simulink library "DigitalControlLib"  (R2017b)
settings: Solver=VariableStepAuto  StartTime=0.0  StopTime=10.0  RelTol=1e-3
settings Model: Creator=alexandersoussan  LastModifiedBy=alexandersoussan

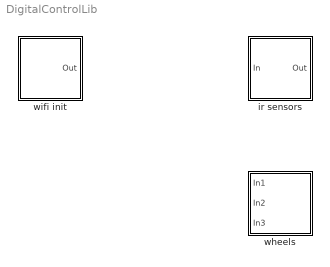
== system DigitalControlLib ==
  ir sensors : Subsystem
  wheels : Subsystem
  wifi init : Subsystem

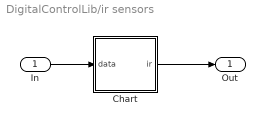
== system DigitalControlLib/ir sensors ==
  In : Inport
  Chart : Stateflow chart  TreatAsAtomicUnit=on
  Out : Outport
  wires:
  Chart/1(ir) -> Out/1
  In/1 -> Chart/1(data)

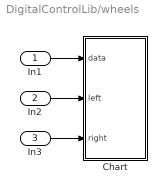
== system DigitalControlLib/wheels ==
  In1 : Inport
  In2 : Inport  Port=2
  In3 : Inport  Port=3
  Chart : Stateflow chart  TreatAsAtomicUnit=on
  wires:
  In1/1 -> Chart/1(data)
  In2/1 -> Chart/2(left)
  In3/1 -> Chart/3(right)

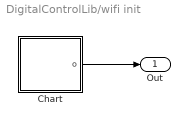
== system DigitalControlLib/wifi init ==
  Chart : Stateflow chart  TreatAsAtomicUnit=on
  Out : Outport
  wires:
  Chart/1(o) -> Out/1

== stateflow chart DigitalControlLib/ir sensors/Chart ==
  state RANGE
    en,du:
    ir=irv;
  (default) -> RANGE
  data: y function_output; ir output; data input
  function y = irv:
    | function y = irv
    | y = [0,0,0,0,0,0];
    | persistent obj
    | coder.extrinsic('evalin')
    | coder.extrinsic('get')
    | coder.extrinsic('RangeStateRoomba')
    | if isempty(obj)
    |     obj = evalin('base','objWs')
    | end
    | coder.extrinsic('RangeStateRoomba')
    | y = RangeStateRoomba(obj);

== stateflow chart DigitalControlLib/wheels/Chart ==
  state Wheels
    en,du:
    wheel(right,left);
  (default) -> Wheels
  data: u1 function_input; u2 function_input; data input; left input; right input
  function wheel(u1,u2):
    | function wheel(u1,u2)
    | persistent obj
    | coder.extrinsic('evalin')
    | coder.extrinsic('get')
    | if isempty(obj)
    |     obj = evalin('base','objWs');
    | end
    | coder.extrinsic('SetWheelVelRoomba')
    | SetWheelVelRoomba(obj,u1,u2);

== stateflow chart DigitalControlLib/wifi init/Chart ==
  state INIT
    en,du:
    tcpInit;
    o=1;
  (default) -> INIT
  data: o output
  function tcpInit:
    | function tcpInit
    | coder.extrinsic('RoombaWifiInit');
    | coder.extrinsic('assignin');
    | persistent obj
    | if isempty(obj)
    | obj = RoombaWifiInit('10.0.0.1','full');
    | assignin('base','objWs', obj);
    | end
